simulink model "IM_model_final"  (R2021a)
settings: Solver=FixedStepAuto  StartTime=0.0  StopTime=10  FixedStep=1e-5  RelTol=1e-3
InitFcn:
  | %% Values of Parameters
  | R1a=0.001579662;
  | R2a=0.001130053590568;
  | X1a=0.0253956;
  | X2a=0.024186280814577;
  | Xma=0.744789315664148;
  | Rca=45.967698519515480;
  | 
  | %% Other Parameters
  | Power=4300e3;
  | Torque=34500;
  | pole=6;
  | pp=pole/2;
  | Vll=700;
  | f=60;
  | Jm=242.28;
  | 
  | 
  | %% Inductances
  | L1a=X1a/2/pi/f;
  | L2a=X2a/2/pi/f;
  | Lma=Xma/2/pi/f;
libraries: spsACVoltageSourceLib x3, spsSeriesRLCBranchLib x3, spsGroundLib x1, spsAsynchronousMachineSIUnitsLib x1, spsMeanLib x1, spsRMSLib x1, spspowerguiLib x1
settings Model: Creator=enes_  LastModifiedBy=enes_

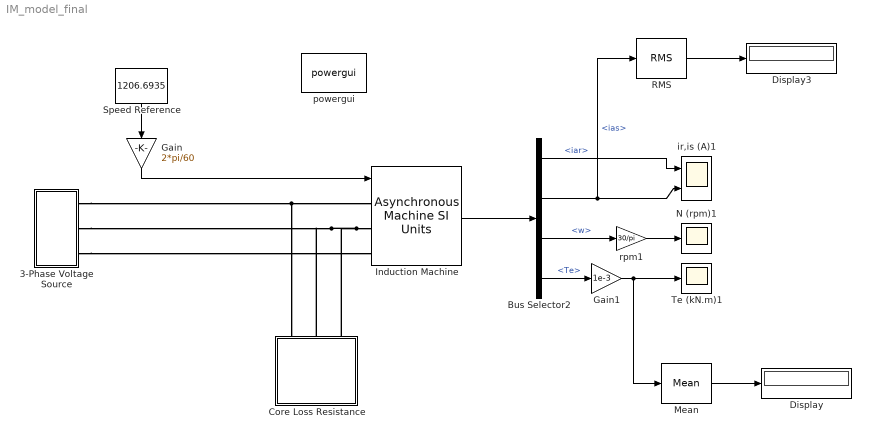
== system IM_model_final ==
  3-Phase Voltage Source : Subsystem
  Bus Selector2 : BusSelector  OutputSignals=iar,ias,w,Te
  Core Loss Resistance : Subsystem
  Display : Display
  Display3 : Display
  Gain : Gain  Gain=2*pi/60
  Gain1 : Gain  Gain=1e-3
  Induction Machine : spsAsynchronousMachineSIUnitsLib/Asynchronous Machine SI Units  RotorType=Squirrel-cage  PresetModel=No  MechanicalLoad=Speed w  ShowDetailedParameters=on  ReferenceFrame=Stationary  Units=SI  MeasurementBus=on  NominalParameters=[Power/2 Vll f]  VoltageRatio=1  Stator=[R1a L1a]  Rotor=[R2a L2a]  Cage1=[ 0.022 0.226/377]  Cage2=[ 0.022 0.226/377]  Lm=Lma  Mechanical=[Jm 0 pp]  PolePairs=pp  InitialConditions="[ 1,0   0,0,0   0,0,0 ]"  SimulateSaturation=off  Saturation=[14.03593122, 27.81365428, 53.79336849, 72.68890987, 97.98006896, 148.6815601, 215.7428561, 302.9841135, 428.7778367 ; 230, 322, 414, 460, 506, 552, 598, 644, 690]  LoadFlowParameters=0  TsPowergui=0  TsBlock=-1  IterativeModel=Trapezoidal non iterative  IterativeDiscreteModel=Trapezoidal non iterative  Pmec=0
      settings: AttributesFormatString=\n
  Mean : spsMeanLib/Mean  Freq=60  Vinit=0  Ts=0
  N (rpm)1 : Scope
  RMS : spsRMSLib/RMS  TrueRMS=off  Freq=60  RMSInit=0  Ts=0
  Speed Reference : Constant  Value=1206.6935
  Te (kN.m)1 : Scope
  ir,is (A)1 : Scope  NumInputPorts=2
  powergui : spspowerguiLib/powergui  SimulationMode=Continuous  SampleTime=0  frequency=60  Iterations=50  frequencyindice=60  Pbase=100e6  ErrMax=1e-4  UnitsV=kV  UnitsW=MW  buscounter=0  FunctionMessages=off  echomessages=off  EnableUseOfTLC=off  CurrentSourceSwitches=off  DisableSnubberDevices=off  DisableRonSwitches=off  DisableVfSwitches=off  DisplayEquations=off  AutomaticDiscreteSolvers=off  SolverType=Tustin  Interpol=off  ExternalGateDelay=off  methode=off  Ts=0  x0status=blocks  SPID=on  SwTol=0  HookPort=off  NonlinearTolerance=1e-4  nMaxIteration=100  ContinueOnMaxIteration=off  RestoreLinks=warning  ResistiveCurrentMeasurement=off  Frange=[0:2:500]  Ylog=off  Xlog=on  ShowGrid=off  save=off  variable=ZData  structure=0  ZoomFFT=on  StartTime=0.0  cycles=1  DisplayStyle=1  fundamental=60  FreqAxis=off  MaxFrequency=1000  frequencyindicesteady=1  RmsSteady=1  display=off
  rpm1 : Gain  Gain=30/pi  SaturateOnIntegerOverflow=on  OutDataTypeStr=Inherit: Same as input  ParamDataTypeStr=Inherit: Same as input
  wires:
  Gain1/1 -> Mean/1, Te (kN.m)1/1
  Bus Selector2/2 -> RMS/1, ir,is (A)1/2  "<ias>"
  rpm1/1 -> N (rpm)1/1
  Bus Selector2/1 -> ir,is (A)1/1  "<iar>"
  Bus Selector2/4 -> Gain1/1  "<Te>"
  Induction Machine/1 -> Bus Selector2/1
  Bus Selector2/3 -> rpm1/1  "<w>"
  Gain/1 -> Induction Machine/1
  Speed Reference/1 -> Gain/1
  Mean/1 -> Display/1
  RMS/1 -> Display3/1
  connections:
  Induction Machine/LConn2 -- 3-Phase Voltage Source/RConn2 -- Core Loss Resistance/LConn2 -- Core Loss Resistance/LConn3
  3-Phase Voltage Source/RConn3 -- Induction Machine/LConn3
  3-Phase Voltage Source/RConn1 -- Induction Machine/LConn1 -- Core Loss Resistance/LConn1

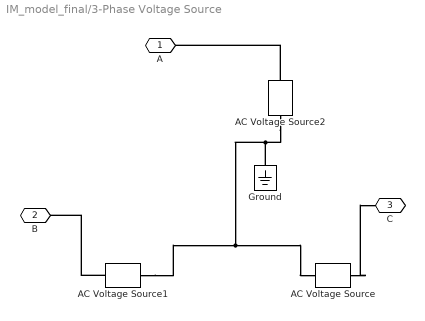
== system IM_model_final/3-Phase Voltage Source ==
  AC Voltage Source : spsACVoltageSourceLib/AC Voltage Source  Amplitude=Vll/sqrt(3)*sqrt(2)  Phase=120  Frequency=f  SampleTime=0  Measurements=None  BusType=swing  Pref=10e3  Qref=0  Qmin=-inf  Qmax=+inf
  AC Voltage Source1 : spsACVoltageSourceLib/AC Voltage Source  Amplitude=Vll/sqrt(3)*sqrt(2)  Phase=240  Frequency=f  SampleTime=0  Measurements=None  BusType=swing  Pref=10e3  Qref=0  Qmin=-inf  Qmax=+inf
  AC Voltage Source2 : spsACVoltageSourceLib/AC Voltage Source  Amplitude=Vll/sqrt(3)*sqrt(2)  Phase=0  Frequency=f  SampleTime=0  Measurements=None  BusType=swing  Pref=10e3  Qref=0  Qmin=-inf  Qmax=+inf
  Ground : spsGroundLib/Ground  LConnTagsString=a
  A : PMIOPort  Side=Right
  B : PMIOPort  Port=2  Side=Right
  C : PMIOPort  Port=3  Side=Right
  connections:
  AC Voltage Source2/LConn1 -- AC Voltage Source1/LConn1 -- AC Voltage Source/LConn1 -- Ground/LConn1
  AC Voltage Source1/RConn1 -- B/RConn1
  AC Voltage Source2/RConn1 -- A/RConn1
  AC Voltage Source/RConn1 -- C/RConn1

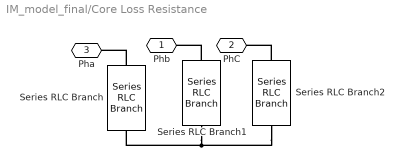
== system IM_model_final/Core Loss Resistance ==
  Series RLC Branch : spsSeriesRLCBranchLib/Series RLC Branch  LConnTagsString=__new0  RConnTagsString=__new0  BranchType=R  Resistance=Rca  Inductance=1e-3  SetiL0=off  InitialCurrent=0  Capacitance=1e-6  Setx0=off  InitialVoltage=0  Measurements=None
  Series RLC Branch1 : spsSeriesRLCBranchLib/Series RLC Branch  LConnTagsString=__new0  RConnTagsString=__new0  BranchType=R  Resistance=Rca  Inductance=1e-3  SetiL0=off  InitialCurrent=0  Capacitance=1e-6  Setx0=off  InitialVoltage=0  Measurements=None
  Series RLC Branch2 : spsSeriesRLCBranchLib/Series RLC Branch  LConnTagsString=__new0  RConnTagsString=__new0  BranchType=R  Resistance=Rca  Inductance=1e-3  SetiL0=off  InitialCurrent=0  Capacitance=1e-6  Setx0=off  InitialVoltage=0  Measurements=None
  Phb : PMIOPort  Side=Left
  PhC : PMIOPort  Port=2  Side=Left
  Pha : PMIOPort  Port=3  Side=Left
  connections:
  Series RLC Branch2/RConn1 -- Series RLC Branch1/RConn1 -- Series RLC Branch/RConn1
  Series RLC Branch/LConn1 -- Pha/RConn1
  Series RLC Branch1/LConn1 -- Phb/RConn1
  Series RLC Branch2/LConn1 -- PhC/RConn1
